simulink model "YAW_tf"  (R2023b)
settings: Solver=FixedStepAuto  StartTime=0  StopTime=t(end)  FixedStep=0.002  RelTol=1e-3
settings Model: Creator=franc  LastModifiedBy=franc

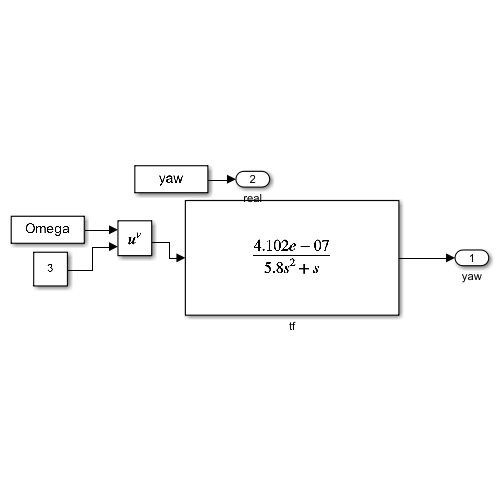
[thumbnail: Simulink's stored preview of the top-level diagram]
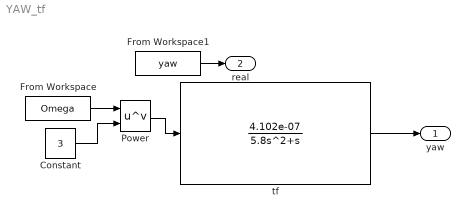
== system YAW_tf ==
  Constant : Constant  Value=3
  From Workspace : FromWorkspace  VariableName=Omega  SampleTime=0.002
  From Workspace1 : FromWorkspace  VariableName=yaw
  Power : Math  Operator=pow
  tf : TransferFcn  Numerator=4.102e-07  Denominator=[5.8 1 0]
  yaw : Outport
  real : Outport  Port=2
  wires:
  Constant/1 -> Power/2
  From Workspace/1 -> Power/1
  Power/1 -> tf/1
  From Workspace1/1 -> real/1
  tf/1 -> yaw/1
